simulink model "PIDController"  (R2018b)
settings: Solver=ode45  StartTime=0.0  StopTime=t_sim  RelTol=1e-5
undefined symbols (not defined in the file): A1, A2, g, h10, h20, Kh, Ki, Km, Kpid, Kv, qu0, Tv, u0
settings Model: Creator=Mislav  LastModifiedBy=student

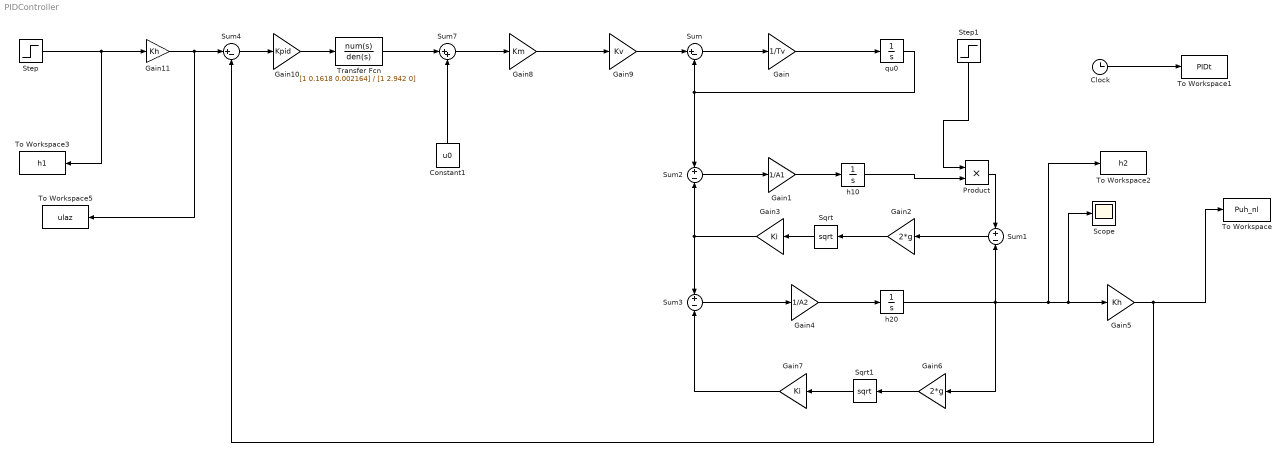
== system PIDController ==
  Clock : Clock
  Constant1 : Constant  Value=u0
  Gain : Gain  Gain=1/Tv
  Gain1 : Gain  Gain=1/A1
  Gain10 : Gain  Gain=Kpid
  Gain11 : Gain  Gain=Kh
  Gain2 : Gain  Gain=2*g
  Gain3 : Gain  Gain=Ki
  Gain4 : Gain  Gain=1/A2
  Gain5 : Gain  Gain=Kh
  Gain6 : Gain  Gain=2*g
  Gain7 : Gain  Gain=Ki
  Gain8 : Gain  Gain=Km
  Gain9 : Gain  Gain=Kv
  Product : Product
  Scope : Scope
  Sqrt : Sqrt  SaturateOnIntegerOverflow=on
  Sqrt1 : Sqrt  SaturateOnIntegerOverflow=on
  Step : Step  Time=100  Before=h20  After=h20*1.1  SampleTime=0
  Step1 : Step  Time=900  Before=1  After=1.02  SampleTime=0
  Sum : Sum  Inputs=|+-
  Sum1 : Sum  Inputs=+-
  Sum2 : Sum  Inputs=+|-
  Sum3 : Sum  Inputs=+|-
  Sum4 : Sum  Inputs=|+-
  Sum7 : Sum  Inputs=|++
  To Workspace : ToWorkspace  VariableName=Puh_nl  SampleTime=-1
      settings: Save2DSignal=2-D array (concatenate along first dimension)
  To Workspace1 : ToWorkspace  VariableName=PIDt  SampleTime=-1
      settings: Save2DSignal=2-D array (concatenate along first dimension)
  To Workspace2 : ToWorkspace  VariableName=h2  SampleTime=-1
      settings: Save2DSignal=2-D array (concatenate along first dimension)
  To Workspace3 : ToWorkspace  VariableName=h1  SampleTime=-1
      settings: Save2DSignal=2-D array (concatenate along first dimension)
  To Workspace5 : ToWorkspace  VariableName=ulaz  SampleTime=-1
      settings: Save2DSignal=2-D array (concatenate along first dimension)
  Transfer Fcn : TransferFcn  Numerator=[1 0.1618 0.002164]  Denominator=[1 2.942 0]
  "h10 " : Integrator  InitialCondition=h10
  "h20 " : Integrator  InitialCondition=h20
  "qu0 " : Integrator  InitialCondition=qu0
  wires:
  Gain4/1 -> "h20 "/1
  Sum7/1 -> Gain8/1
  Sqrt/1 -> Gain3/1
  Constant1/1 -> Sum7/2
  Sum4/1 -> Gain10/1
  Sum1/1 -> Gain2/1
  Gain2/1 -> Sqrt/1
  Sqrt1/1 -> Gain7/1
  Gain7/1 -> Sum3/2
  Step/1 -> Gain11/1, To Workspace3/1
  Gain5/1 -> To Workspace/1, Sum4/2
  Gain3/1 -> Sum2/2, Sum3/1
  "qu0 "/1 -> Sum/2, Sum2/1
  Sum/1 -> Gain/1
  Sum3/1 -> Gain4/1
  "h20 "/1 -> Gain6/1, To Workspace2/1, Scope/1, Gain5/1, Sum1/2
  Gain1/1 -> "h10 "/1
  Gain11/1 -> Sum4/1, To Workspace5/1
  Sum2/1 -> Gain1/1
  Gain/1 -> "qu0 "/1
  Gain6/1 -> Sqrt1/1
  Clock/1 -> To Workspace1/1
  Gain9/1 -> Sum/1
  Gain8/1 -> Gain9/1
  "h10 "/1 -> Product/2
  Step1/1 -> Product/1
  Product/1 -> Sum1/1
  Gain10/1 -> Transfer Fcn/1
  Transfer Fcn/1 -> Sum7/1
